simulink model "Golf_Cart_Supervisory_Controller"  (R2019b)
settings: Solver=FixedStepAuto  StartTime=0.0  StopTime=5  FixedStep=0.01  RelTol=1e-3  EnableMultiTasking=on
PreLoadFcn:
  | load exampleMap
  | 
  | scanAngles = [-3*pi/8;-pi/4;-pi/8;0;pi/8;pi/4;3*pi/8];
  | maxRange = 6;
  | 
  | sampleTime = 0.05;
libraries: mobileRoboticsLib x3, simulink x1
settings Model: NumberOfSteps=100  EnablePacing=on  PacingRate=0.010000  Creator=scastro  LastModifiedBy=shree
settings SolverCC: AutoInsertRateTranBlk=on
settings DataIOCC: LimitDataPoints=on  ReturnWorkspaceOutputs=off
settings OptimizationCC: LifeSpan=inf
settings DebuggingCC: AllowSymbolicDim=off  PregeneratedLibrarySubsystemCodeDiagnostic=none  SFUnexpectedBacktrackingDiag=warning  SFNoUnconditionalDefaultTransitionDiag=warning  SFExecutionAtInitializationDiag=none  ArithmeticOperatorsInVariantConditions=warning
settings SFSimCC: SimUseLocalCustomCode=off  CustomCodeUndefinedFunction=UseInterfaceOnly
settings RTWCC: RTWUseLocalCustomCode=off
settings CodeAppCC: StateflowObjectComments=on
settings GRTTargetCC: TargetLangStandard=C89/C90 (ANSI)  GeneratePreprocessorConditionals=Disable all
settings ConfigComp: CovMetricSettings=dw  CovHtmlReporting=on  CovSaveCumulativeToWorkspaceVar=on  CovSaveSingleToWorkspaceVar=on  CovExternalEMLEnable=off  CovSFcnEnable=off
settings SimscapeCC: SimscapeNominalValues="[{\"value\":\"10\",\"unit\":\"V\"},{\"value\":\"1\",\"unit\":\"A\"},{\"value\":\"10\",\"unit\":\"N*m\"},{\"value\":\"10\",\"unit\":\"bar\"},{\"value\":\"100\",\"unit\":\"kJ/kg\"},{\"value\":\"1\",\"unit\":\"kW\"},{\"value\":\"300\",\"unit\":\"K\"},{\"value\":\"100\",\"unit\":\"cm^3/s\"},{\"value\":\"1\",\"unit\":\"kN\"},{\"value\":\"1\",\"unit\":\"g/cm^3\"},{\"value\":\"1\",\"unit\":\"l\"},{\"value\":\"1\",\"unit\":\"cm^2\"},{\"value\":\"60\",\"unit\":\"Hz\"}]"  SimscapeLogType=all  SimscapeLogDataHistory=10000
settings ConfigurationSet: Description=SimMechanics 2G
settings ExplorerConfigSet: InternalSimMechanicsExplorerSettings="<ExplorerConfiguration><canonicalview>default</canonicalview><AnimationSetting><BasePlaybackSpeed>1.0</BasePlaybackSpeed><PlaybackSpeedFactor>1.0</PlaybackSpeedFactor></AnimationSetting><TilePanel><TileInfo><Tiles Columns=\"1\" Count=\"1\" Rows=\"1\"><Column Weight=\"1\"/><Row Weight=\"1\"/><Tile Height=\"1\" Width=\"1\" X=\"0\" Y=\"0\"/></Tiles></TileInfo><SceneInfo><SceneViewer><BGColor><R>0.60000002384185791</R><G>0.60000002384185791</G><B>0.60000002384185791</B></BGColor><Camera><DoPerspective>off</DoPerspective><Position><X>-1.70656042355848525</X><Y>-0.974920623359631922</Y><Z>4.72930454537082046</Z></Position><Center><X>0.552860638431633689</X><Y>1.42025063411503494</Y><Z>1.4843509506914252</Z></Center><Up><X>0.664249622453917166</X><Y>0.300615402055903091</Y><Z>0.684399604848363485</Z></Up><ViewLimDist>1</ViewLimDist><YLim>2.77881717169207398</YLim><XLim>3.55928742670435394</XLim></Camera></SceneViewer></SceneInfo></TilePanel><MechEditorPanel><Cameras/><GfxPanelCameraMap/><VideoCreator><PlaybackSpeedRatio>1.0</PlaybackSpeedRatio><FrameRate>30</FrameRate><VideoFormat>Motion JPEG AVI</VideoFormat><FrameSize>auto</FrameSize></VideoCreator></MechEditorPanel></ExplorerConfiguration>"

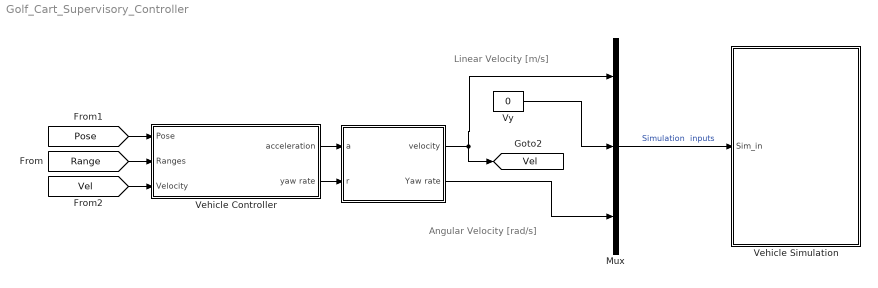
== system Golf_Cart_Supervisory_Controller ==
  note: Linear Velocity [m/s]
  note: Angular Velocity [rad/s]
  " " : Subsystem
  Mux : Mux  Inputs=3
  Vehicle Controller : Subsystem
  Vehicle Simulation : Subsystem
  Vy : Constant  Value=0
  tag scope: Vel=global
  wires:
  Vy/1 -> Mux/2
  [Pose] -> Vehicle Controller/1(Pose)
  [Range] -> Vehicle Controller/2(Ranges)
  " "/2(Yaw rate) -> Mux/3
  " "/1(velocity) -> Mux/1, [Vel]
  [Vel] -> Vehicle Controller/3(Velocity)
  Vehicle Controller/1("acceleration ") -> " "/1(a)
  Vehicle Controller/2("yaw rate ") -> " "/2(r)
  Mux/1 -> Vehicle Simulation/1(Sim_in)  "Simulation  inputs"

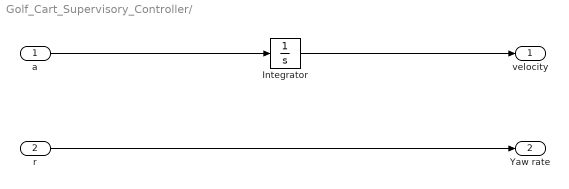
== system Golf_Cart_Supervisory_Controller/  ==
  a : Inport
  r : Inport  Port=2
  Integrator : Integrator  InitialCondition=2  LimitOutput=on  UpperSaturationLimit=3.2  LowerSaturationLimit=-3.2
  velocity : Outport
  Yaw rate : Outport  Port=2
  wires:
  a/1 -> Integrator/1
  Integrator/1 -> velocity/1
  r/1 -> Yaw rate/1

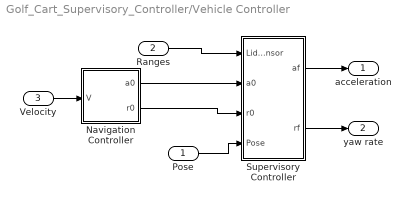
== system Golf_Cart_Supervisory_Controller/Vehicle Controller ==
  Pose : Inport
  Ranges : Inport  Port=2
  Velocity : Inport  Port=3
  Navigation Controller : Subsystem
  Supervisory Controller : Subsystem
  "acceleration " : Outport
  "yaw rate " : Outport  Port=2
  wires:
  Velocity/1 -> Navigation Controller/1(V)
  Ranges/1 -> Supervisory Controller/1(Lidar_Sensor)
  Pose/1 -> Supervisory Controller/4(Pose)
  Navigation Controller/1(a0) -> Supervisory Controller/2(a0)
  Navigation Controller/2(r0) -> Supervisory Controller/3(r0)
  Supervisory Controller/1(af) -> "acceleration "/1
  Supervisory Controller/2(rf) -> "yaw rate "/1

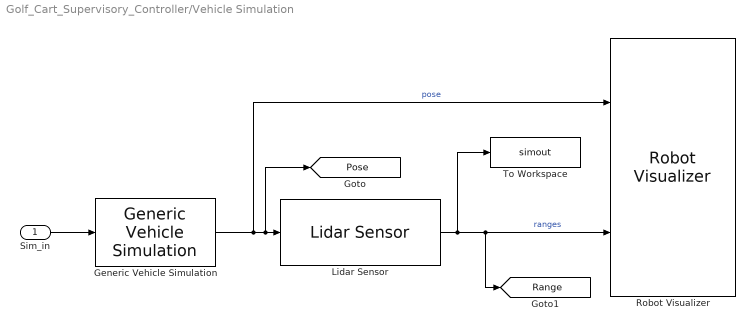
== system Golf_Cart_Supervisory_Controller/Vehicle Simulation ==
  Sim_in : Inport
  Generic Vehicle Simulation : mobileRoboticsLib/Utilities/Generic Vehicle Simulation  initX=3  initY=4  initAngle=0  Ts=sampleTime
      settings: SourceProductName=Mobile Robotics Simulation Toolbox
  Lidar Sensor : mobileRoboticsLib/Environments/Lidar Sensor  mapName=map  sensorOffset=[ 0 0 ]  scanAngles=scanAngles  maxRange=maxRange
      settings: SourceProductName=Mobile Robotics Simulation Toolbox
  Robot Visualizer : mobileRoboticsLib/Environments/Robot Visualizer  Priority=99  robotRadius=0  mapName=map  showTrajectory=on  hasWaypoints=off  hasLidar=on  sensorOffset=[ 0 0 ]  scanAngles=scanAngles  hasObjDetector=off  objDetectorOffset=[ 0, 0 ]  objDetectorAngle=0  objDetectorFOV=pi/4  objDetectorMaxRange=5  objectColors=[ 1, 0, 0; 0, 1, 0; 0, 0, 1 ]  objectMarkers='s'
  To Workspace : ToWorkspace  VariableName=simout  SampleTime=-1
  tag scope: Pose=global, Range=global
  wires:
  Generic Vehicle Simulation/1 -> Robot Visualizer/1, [Pose], Lidar Sensor/1  "pose"
  Lidar Sensor/1 -> To Workspace/1, [Range], Robot Visualizer/2  "ranges"
  Sim_in/1 -> Generic Vehicle Simulation/1

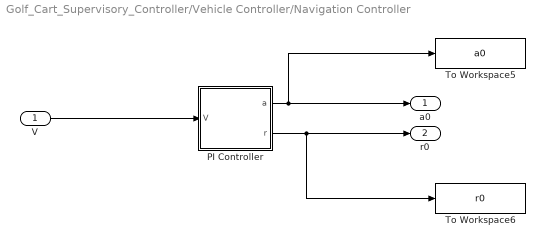
== system Golf_Cart_Supervisory_Controller/Vehicle Controller/Navigation Controller ==
  V : Inport
  PI Controller : Subsystem
  To Workspace5 : ToWorkspace  VariableName=a0  SaveFormat=Structure  SampleTime=-1
  To Workspace6 : ToWorkspace  VariableName=r0  SaveFormat=Structure  SampleTime=-1
  a0 : Outport
  r0 : Outport  Port=2
  wires:
  PI Controller/2(r) -> r0/1, To Workspace6/1
  PI Controller/1(a) -> a0/1, To Workspace5/1
  V/1 -> PI Controller/1(V)

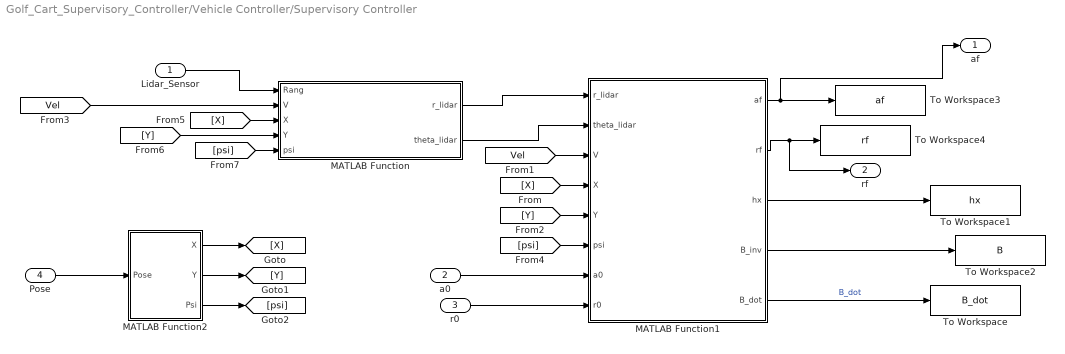
== system Golf_Cart_Supervisory_Controller/Vehicle Controller/Supervisory Controller ==
  Lidar_Sensor : Inport
  a0 : Inport  Port=2
  r0 : Inport  Port=3
  Pose : Inport  Port=4
  MATLAB Function : MATLAB Function  TreatAsAtomicUnit=on
  MATLAB Function1 : MATLAB Function  TreatAsAtomicUnit=on
  MATLAB Function2 : MATLAB Function  TreatAsAtomicUnit=on
  To Workspace : ToWorkspace  VariableName=B_dot  SaveFormat=Structure  SampleTime=-1
  To Workspace1 : ToWorkspace  VariableName=hx  SaveFormat=Structure  SampleTime=-1
  To Workspace2 : ToWorkspace  VariableName=B  SaveFormat=Structure  SampleTime=-1
  To Workspace3 : ToWorkspace  VariableName=af  SaveFormat=Structure  SampleTime=-1
  To Workspace4 : ToWorkspace  VariableName=rf  SaveFormat=Structure  SampleTime=-1
  af : Outport
  rf : Outport  Port=2
  wires:
  MATLAB Function1/3(hx) -> To Workspace1/1
  MATLAB Function1/2(rf) -> rf/1, To Workspace4/1
  MATLAB Function1/1(af) -> af/1, To Workspace3/1
  r0/1 -> MATLAB Function1/8(r0)
  MATLAB Function1/5(B_dot) -> To Workspace/1  "B_dot"
  a0/1 -> MATLAB Function1/7(a0)
  Lidar_Sensor/1 -> MATLAB Function/1(Rang)
  MATLAB Function1/4(B_inv) -> To Workspace2/1
  Pose/1 -> MATLAB Function2/1(Pose)
  MATLAB Function2/1(X) -> [X]
  MATLAB Function2/2(Y) -> [Y]
  MATLAB Function2/3(Psi) -> [psi]
  MATLAB Function/1(r_lidar) -> MATLAB Function1/1(r_lidar)
  MATLAB Function/2(theta_lidar) -> MATLAB Function1/2(theta_lidar)
  [Vel] -> MATLAB Function/2(V)
  [Vel] -> MATLAB Function1/3(V)
  [X] -> MATLAB Function1/4(X)
  [Y] -> MATLAB Function1/5(Y)
  [psi] -> MATLAB Function1/6(psi)
  [X] -> MATLAB Function/3(X)
  [Y] -> MATLAB Function/4(Y)
  [psi] -> MATLAB Function/5(psi)

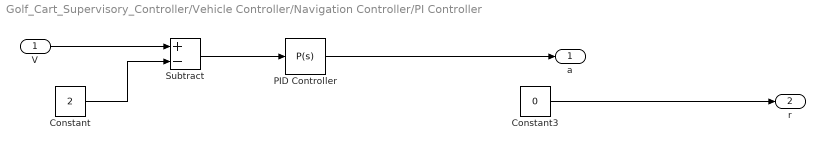
== system Golf_Cart_Supervisory_Controller/Vehicle Controller/Navigation Controller/PI Controller ==
  V : Inport
  Constant : Constant  Value=2
  Constant3 : Constant  Value=0
  PID Controller : simulink/Continuous/PID Controller  Controller=P  Form=Parallel  TimeDomain=Continuous-time  SampleTime=-1  IntegratorMethod=Forward Euler  FilterMethod=Forward Euler  ControllerParametersSource=internal  P=-1/0.05  I=1  D=0  UseFilter=on  N=100  TunerSelectOption=Transfer Function Based (PID Tuner App)  InitialConditionSource=internal  InitialConditionForIntegrator=0  InitialConditionForFilter=0  DifferentiatorICPrevScaledInput=0  ExternalReset=none  TrackingMode=off  Kt=1  LimitOutput=on  UpperSaturationLimit=4  LowerSaturationLimit=-4  LinearizeAsGain=on  AntiWindupMode=none  Kb=1  POutMin=[]  POutMax=[]  IOutMin=[]  IOutMax=[]  DOutMin=[]  DOutMax=[]  NOutMin=[]  NOutMax=[]  SumOutMin=[]  SumOutMax=[]  SaturationOutMin=[]  SaturationOutMax=[]  PParamMin=[]  PParamMax=[]  IParamMin=[]  IParamMax=[]  DParamMin=[]  DParamMax=[]  NParamMin=[]  NParamMax=[]  KbParamMin=[]  KbParamMax=[]  KtParamMin=[]  KtParamMax=[]  KbOutMin=[]  KbOutMax=[]  KtOutMin=[]  KtOutMax=[]  IntegratorOutMin=[]  IntegratorOutMax=[]  FilterOutMin=[]  FilterOutMax=[]  SumI1OutMin=[]  SumI1OutMax=[]  SumI2OutMin=[]  SumI2OutMax=[]  SumI3OutMin=[]  SumI3OutMax=[]  SumI4OutMin=[]  SumI4OutMax=[]  SumDOutMin=[]  SumDOutMax=[]  DifferentiatorOutMin=[]  DifferentiatorOutMax=[]  FilterDiffOutCoefMin=[]  FilterDiffOutCoefMax=[]  ReciprocalOutMin=[]  ReciprocalOutMax=[]  SumDenOutMin=[]  SumDenOutMax=[]  SumNumOutMin=[]  SumNumOutMax=[]  DivideOutMin=[]  DivideOutMax=[]  IntegratorContinuousStateAttributes=''  IntegratorStateMustResolveToSignalObject=off  IntegratorRTWStateStorageClass=Auto  FilterContinuousStateAttributes=''  FilterStateMustResolveToSignalObject=off  FilterRTWStateStorageClass=Auto  ParallelPVariant=InternalParameters  IdealPVariant=Disabled  IVariant=Disabled  DVariant=Disabled  IntegratorVariant=Disabled  SatVariant=Enabled  AWVariant=Disabled  PCopyVariant=Disabled  TRVariant=Disabled  FdbkBlocksVariant=Forward  IdealPFdbkVariant=Disabled  SatFdbkVariant=Disabled  DerivativeFilterVariant=Disabled  NVariant=Disabled  NCopyVariant=Disabled_SignalSpec  FilterICVariant=Disabled  IntegratorICVariant=Disabled  ExternalResetVariant=Disabled  TRSumVariant=Passthrough  SumFdbkVariant=Disabled  SumVariant=Passthrough_P
  Subtract : Sum  Inputs=+-
  a : Outport
  r : Outport  Port=2
  wires:
  PID Controller/1 -> a/1
  Constant3/1 -> r/1
  V/1 -> Subtract/1
  Subtract/1 -> PID Controller/1
  Constant/1 -> Subtract/2

== matlab function Golf_Cart_Supervisory_Controller/Vehicle Controller/Supervisory Controller/MATLAB Function1 ==
  data: r_lidar input; theta_lidar input; af output; V input; X input; Y input; psi input; a0 input; r0 input; rf output; hx output; B_inv output; B_dot output
function [af,rf,hx, B_inv, B_dot] = fcn(r_lidar, theta_lidar, V, X, Y, psi, a0, r0)
bx = X + r_lidar * cos(psi+theta_lidar);
by = Y + r_lidar * sin(psi+theta_lidar);
z_safe = 0.8;
Ts = 0.5;
p1 = (bx - X - V * Ts * cos(psi));
p2 = (by - Y - V * Ts * sin(psi));
hx = ((p1^2 + p2^2)^0.5);

B = 1/(hx - z_safe);
%B = -log(hx-z_safe);
p3 = (-V * (p1 * cos(psi) + p2 * sin(psi)))/hx;
p4 = (V * Ts * (p1 * sin(psi) - p2 * cos(psi)))/hx;
p5 = (-Ts * (p1 * cos(psi) + p2 * sin(psi)))/hx;
%Gamma = 4.15*10^9;
%Gamma = 31.5*0+10^4;
Gamma =5.15*10^7;
 A = [-p5,-p4];
 b = p3 + (Gamma / B^3);

%A = [-p5,-p4];
%b = p3 + Gamma * (hx-z_safe) / B;

y0=[a0,r0];
fun = @(y)(y-y0)*[1,0;0,1]*(y-y0)';

options = optimoptions('fmincon','Display','iter','Algorithm','sqp-legacy');
K = fmincon(fun,y0,A,b,[],[],[-4,-5],[0,5],[],options);
    
af = K(1);
rf = K(2);
 
B_inv=Gamma/B;
B_dot=(-p3-p4*rf-p5*af)*B^2;
ctrl=B_dot-Gamma/B;
end

== matlab function Golf_Cart_Supervisory_Controller/Vehicle Controller/Supervisory Controller/MATLAB Function ==
  data: Rang input; r_lidar output; theta_lidar output; V input; X input; Y input; psi input
function [r_lidar,theta_lidar] = fcn(Rang, V, X, Y, psi)

z_safe = 0.8;
Ts = 0.5;
scanAngles=linspace(-pi/2,pi/2,101);

%lidars=lidarScan(Rang,scanAngles);
%lidarpos=lidars.Cartesian;
[pks,locs]=min(Rang);
r_lidar=pks;
% % dX=pks*cos(scanAngles(locs));
% % dY=pks*sin(scanAngles(locs));
theta_lidar=scanAngles(locs);
hmax=10;
for i=1:length(Rang)
    bx = X + Rang(i) * cos(psi+scanAngles(i));
    by = Y + Rang(i) * sin(psi+scanAngles(i));
    p1 = (bx - X - V * Ts * cos(psi));
    p2 = (by - Y - V * Ts * sin(psi));
    hx = ((p1^2 + p2^2)^0.5);
    if hx<=hmax
        locs=i;
        hmax=hx;
    end
end
theta_lidar=scanAngles(locs);
r_lidar=Rang(locs);

== matlab function Golf_Cart_Supervisory_Controller/Vehicle Controller/Supervisory Controller/MATLAB Function2 ==
  data: X output; Y output; Pose input; Psi output
function [X,Y,Psi]  = fcn(Pose)
X=Pose(1);
Y=Pose(2);
Psi=Pose(3);
